simulink model "Per_MKM"  (R2019a)
settings: Solver=FixedStepDiscrete  StartTime=0.0  StopTime=50  FixedStep=1  RelTol=1e-3
undefined symbols (not defined in the file or in its folder): ADAS, ADAS_Setting, KeyPress, Setting
libraries: simulink x102
(part 2 of 2)

== system Per_MKM/Seat_POsitioning_Subsystem/POS_Control5/Subsystem4 ==
  In1 : Inport
  Data Store Read14 : DataStoreRead  DataStoreName=POS_M5
  Data Store Read15 : DataStoreRead  DataStoreName=POS_S15
  Data Store Read16 : DataStoreRead  DataStoreName=POS_S25
  Data Type Conversion : DataTypeConversion
  Multiport Switch3 : MultiPortSwitch  DataPortOrder=Zero-based contiguous  DataPortForDefault=Additional data port  zeroidx=on
  Out1 : Outport
  Out2 : Outport  Port=2
  wires:
  Data Store Read16/1 -> Multiport Switch3/4
  Data Store Read15/1 -> Multiport Switch3/3
  Data Type Conversion/1 -> Multiport Switch3/1
  Multiport Switch3/1 -> Out2/1
  Data Store Read14/1 -> Multiport Switch3/2, Multiport Switch3/5
  In1/1 -> Data Type Conversion/1, Out1/1

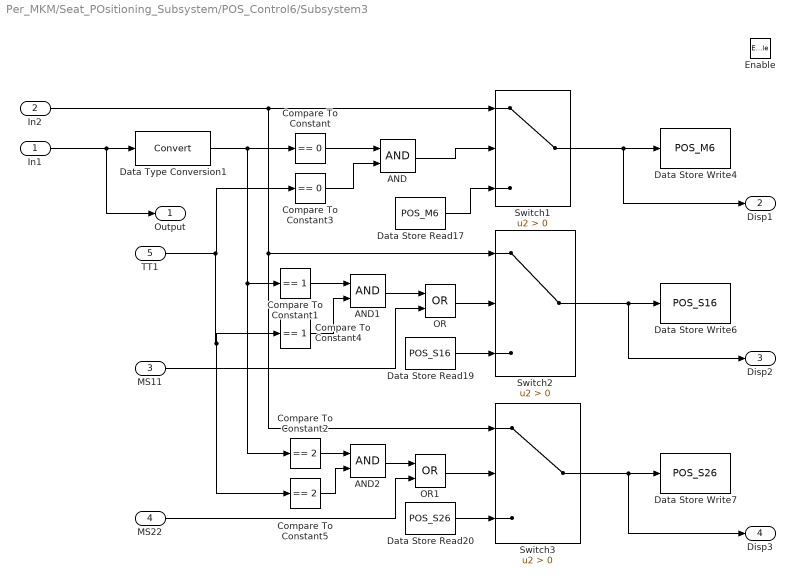
== system Per_MKM/Seat_POsitioning_Subsystem/POS_Control6/Subsystem3 ==
  In1 : Inport
  In2 : Inport  Port=2
  MS11 : Inport  Port=3
  MS22 : Inport  Port=4
  TT1 : Inport  Port=5
  Enable : EnablePort
  AND : Logic  AllPortsSameDT=off  OutDataTypeStr=boolean
  AND1 : Logic  AllPortsSameDT=off  OutDataTypeStr=boolean
  AND2 : Logic  AllPortsSameDT=off  OutDataTypeStr=boolean
  Compare To Constant : simulink/Logic and Bit Operations/Compare To Constant  relop===  const=0  OutDataTypeStr=boolean
  Compare To Constant1 : simulink/Logic and Bit Operations/Compare To Constant  relop===  const=1  OutDataTypeStr=boolean
  Compare To Constant2 : simulink/Logic and Bit Operations/Compare To Constant  relop===  const=2  OutDataTypeStr=boolean
  Compare To Constant3 : simulink/Logic and Bit Operations/Compare To Constant  relop===  const=0  OutDataTypeStr=boolean
  Compare To Constant4 : simulink/Logic and Bit Operations/Compare To Constant  relop===  const=1  OutDataTypeStr=boolean
  Compare To Constant5 : simulink/Logic and Bit Operations/Compare To Constant  relop===  const=2  OutDataTypeStr=boolean
  Data Store Read17 : DataStoreRead  DataStoreName=POS_M6
  Data Store Read19 : DataStoreRead  DataStoreName=POS_S16
  Data Store Read20 : DataStoreRead  DataStoreName=POS_S26
  Data Store Write4 : DataStoreWrite  DataStoreName=POS_M6
  Data Store Write6 : DataStoreWrite  DataStoreName=POS_S16
  Data Store Write7 : DataStoreWrite  DataStoreName=POS_S26
  Data Type Conversion1 : DataTypeConversion
  OR : Logic  Operator=OR  AllPortsSameDT=off  OutDataTypeStr=boolean
  OR1 : Logic  Operator=OR  AllPortsSameDT=off  OutDataTypeStr=boolean
  Switch1 : Switch  Criteria=u2 > Threshold
  Switch2 : Switch  Criteria=u2 > Threshold
  Switch3 : Switch  Criteria=u2 > Threshold
  Output : Outport
  Disp1 : Outport  Port=2
  Disp2 : Outport  Port=3
  Disp3 : Outport  Port=4
  wires:
  Data Type Conversion1/1 -> Compare To Constant/1, Compare To Constant2/1, Compare To Constant1/1
  Switch2/1 -> Disp2/1, Data Store Write6/1
  Data Store Read20/1 -> Switch3/3
  Switch3/1 -> Disp3/1, Data Store Write7/1
  Switch1/1 -> Disp1/1, Data Store Write4/1
  Data Store Read19/1 -> Switch2/3
  Data Store Read17/1 -> Switch1/3
  In1/1 -> Output/1, Data Type Conversion1/1
  In2/1 -> Switch1/1, Switch2/1, Switch3/1
  OR/1 -> Switch2/2
  OR1/1 -> Switch3/2
  MS11/1 -> OR/2
  MS22/1 -> OR1/2
  AND/1 -> Switch1/2
  Compare To Constant/1 -> AND/1
  Compare To Constant3/1 -> AND/2
  TT1/1 -> Compare To Constant5/1, Compare To Constant4/1, Compare To Constant3/1
  Compare To Constant1/1 -> AND1/1
  Compare To Constant4/1 -> AND1/2
  AND1/1 -> OR/1
  AND2/1 -> OR1/1
  Compare To Constant2/1 -> AND2/1
  Compare To Constant5/1 -> AND2/2

== system Per_MKM/Seat_POsitioning_Subsystem/POS_Control6/Subsystem4 ==
  In1 : Inport
  Data Store Read14 : DataStoreRead  DataStoreName=POS_M6
  Data Store Read15 : DataStoreRead  DataStoreName=POS_S16
  Data Store Read16 : DataStoreRead  DataStoreName=POS_S26
  Data Type Conversion : DataTypeConversion
  Multiport Switch3 : MultiPortSwitch  DataPortOrder=Zero-based contiguous  DataPortForDefault=Additional data port  zeroidx=on
  Out1 : Outport
  Out2 : Outport  Port=2
  wires:
  In1/1 -> Out1/1, Data Type Conversion/1
  Data Store Read14/1 -> Multiport Switch3/5, Multiport Switch3/2
  Multiport Switch3/1 -> Out2/1
  Data Type Conversion/1 -> Multiport Switch3/1
  Data Store Read15/1 -> Multiport Switch3/3
  Data Store Read16/1 -> Multiport Switch3/4

== system Per_MKM/Subsystem2/Subsystem/Subsystem_ACC ==
  In1 : Inport
  ACC2 : simulink/Sources/Enumerated Constant  OutDataTypeStr=Enum: ADAS  Value=ADAS.Adaptive_Cruse_Control_Enable  SampleTime=inf
      settings: SourceProductName=Simulink
  ACC3 : simulink/Sources/Enumerated Constant  OutDataTypeStr=Enum: ADAS  Value=ADAS.Adaptive_Cruse_Control_Disable  SampleTime=inf
      settings: SourceProductName=Simulink
  ACC4 : simulink/Sources/Enumerated Constant  OutDataTypeStr=Enum: ADAS  Value=ADAS.Disable  SampleTime=inf
      settings: SourceProductName=Simulink
  Data Store Read1 : DataStoreRead  DataStoreName=ADAS_M
  Data Store Read2 : DataStoreRead  DataStoreName=ADAS_S1
  Data Store Read3 : DataStoreRead  DataStoreName=ADAS_S2
  Data Type Conversion{2..6} (5 alike) : DataTypeConversion
  Enumerated Constant : simulink/Sources/Enumerated Constant  OutDataTypeStr=Enum: KeyPress  Value=KeyPress.No_User  SampleTime=inf
      settings: SourceProductName=Simulink
  Multiport Switch : MultiPortSwitch
  Multiport Switch1 : MultiPortSwitch  DataPortOrder=Zero-based contiguous  Inputs=4  zeroidx=on
  Out1 : Outport
  wires:
  ACC4/1 -> Multiport Switch/4
  Data Store Read3/1 -> Data Type Conversion5/1
  Data Type Conversion4/1 -> Multiport Switch1/3
  ACC3/1 -> Multiport Switch/3
  Data Store Read1/1 -> Data Type Conversion3/1
  Multiport Switch1/1 -> Multiport Switch/1
  ACC2/1 -> Multiport Switch/2
  In1/1 -> Data Type Conversion2/1
  Data Store Read2/1 -> Data Type Conversion4/1
  Enumerated Constant/1 -> Data Type Conversion6/1
  Data Type Conversion2/1 -> Multiport Switch1/1
  Data Type Conversion5/1 -> Multiport Switch1/4
  Data Type Conversion3/1 -> Multiport Switch1/2
  Data Type Conversion6/1 -> Multiport Switch1/5
  Multiport Switch/1 -> Out1/1

== system Per_MKM/Subsystem2/Subsystem/Subsystem_APSD ==
  In1 : Inport
  ACC2 : simulink/Sources/Enumerated Constant  OutDataTypeStr=Enum: ADAS  Value=ADAS.Automatic_Parking_System_Enable  SampleTime=inf
      settings: SourceProductName=Simulink
  ACC3 : simulink/Sources/Enumerated Constant  OutDataTypeStr=Enum: ADAS  Value=ADAS.Automatic_Parking_System_Disable  SampleTime=inf
      settings: SourceProductName=Simulink
  ACC4 : simulink/Sources/Enumerated Constant  OutDataTypeStr=Enum: ADAS  Value=ADAS.Disable  SampleTime=inf
      settings: SourceProductName=Simulink
  Data Store Read1 : DataStoreRead  DataStoreName=ADAS_M2
  Data Store Read2 : DataStoreRead  DataStoreName=ADAS_S12
  Data Store Read3 : DataStoreRead  DataStoreName=ADAS_S22
  Data Type Conversion{2..6} (5 alike) : DataTypeConversion
  Enumerated Constant : simulink/Sources/Enumerated Constant  OutDataTypeStr=Enum: KeyPress  Value=KeyPress.No_User  SampleTime=inf
      settings: SourceProductName=Simulink
  Multiport Switch : MultiPortSwitch
  Multiport Switch1 : MultiPortSwitch  DataPortOrder=Zero-based contiguous  Inputs=4  zeroidx=on
  Out1 : Outport
  wires:
  Data Store Read2/1 -> Data Type Conversion4/1
  ACC2/1 -> Multiport Switch/2
  Enumerated Constant/1 -> Data Type Conversion6/1
  ACC3/1 -> Multiport Switch/3
  Data Type Conversion2/1 -> Multiport Switch1/1
  Data Type Conversion4/1 -> Multiport Switch1/3
  Data Type Conversion6/1 -> Multiport Switch1/5
  Data Store Read3/1 -> Data Type Conversion5/1
  ACC4/1 -> Multiport Switch/4
  Data Type Conversion3/1 -> Multiport Switch1/2
  Data Type Conversion5/1 -> Multiport Switch1/4
  Data Store Read1/1 -> Data Type Conversion3/1
  Multiport Switch1/1 -> Multiport Switch/1
  In1/1 -> Data Type Conversion2/1
  Multiport Switch/1 -> Out1/1

== system Per_MKM/Subsystem2/Subsystem/Subsystem_DDDE ==
  In1 : Inport
  ACC2 : simulink/Sources/Enumerated Constant  OutDataTypeStr=Enum: ADAS  Value=ADAS.Driver_Drowsiness_detection_Enable  SampleTime=inf
      settings: SourceProductName=Simulink
  ACC3 : simulink/Sources/Enumerated Constant  OutDataTypeStr=Enum: ADAS  Value=ADAS.Driver_Drowsiness_detection_Disable  SampleTime=inf
      settings: SourceProductName=Simulink
  ACC4 : simulink/Sources/Enumerated Constant  OutDataTypeStr=Enum: ADAS  Value=ADAS.Disable  SampleTime=inf
      settings: SourceProductName=Simulink
  Data Store Read1 : DataStoreRead  DataStoreName=ADAS_M1
  Data Store Read2 : DataStoreRead  DataStoreName=ADAS_S11
  Data Store Read3 : DataStoreRead  DataStoreName=ADAS_S21
  Data Type Conversion{2..6} (5 alike) : DataTypeConversion
  Enumerated Constant : simulink/Sources/Enumerated Constant  OutDataTypeStr=Enum: KeyPress  Value=KeyPress.No_User  SampleTime=inf
      settings: SourceProductName=Simulink
  Multiport Switch : MultiPortSwitch
  Multiport Switch1 : MultiPortSwitch  DataPortOrder=Zero-based contiguous  Inputs=4  zeroidx=on
  Out1 : Outport
  wires:
  Enumerated Constant/1 -> Data Type Conversion6/1
  Data Store Read3/1 -> Data Type Conversion5/1
  Data Store Read1/1 -> Data Type Conversion3/1
  ACC4/1 -> Multiport Switch/4
  Multiport Switch1/1 -> Multiport Switch/1
  ACC3/1 -> Multiport Switch/3
  Data Type Conversion6/1 -> Multiport Switch1/5
  Data Type Conversion5/1 -> Multiport Switch1/4
  Data Type Conversion3/1 -> Multiport Switch1/2
  Data Type Conversion2/1 -> Multiport Switch1/1
  Data Store Read2/1 -> Data Type Conversion4/1
  Data Type Conversion4/1 -> Multiport Switch1/3
  ACC2/1 -> Multiport Switch/2
  In1/1 -> Data Type Conversion2/1
  Multiport Switch/1 -> Out1/1

== system Per_MKM/Subsystem2/Subsystem/Subsystem_TSRC ==
  In1 : Inport
  ACC2 : simulink/Sources/Enumerated Constant  OutDataTypeStr=Enum: ADAS  Value=ADAS.Trafic_Signal_Recognization_Enable  SampleTime=inf
      settings: SourceProductName=Simulink
  ACC3 : simulink/Sources/Enumerated Constant  OutDataTypeStr=Enum: ADAS  Value=ADAS.Trafic_Signal_Recognization_Disable  SampleTime=inf
      settings: SourceProductName=Simulink
  ACC4 : simulink/Sources/Enumerated Constant  OutDataTypeStr=Enum: ADAS  Value=ADAS.Disable  SampleTime=inf
      settings: SourceProductName=Simulink
  Data Store Read1 : DataStoreRead  DataStoreName=ADAS_M3
  Data Store Read2 : DataStoreRead  DataStoreName=ADAS_S13
  Data Store Read3 : DataStoreRead  DataStoreName=ADAS_S23
  Data Type Conversion{2..6} (5 alike) : DataTypeConversion
  Enumerated Constant : simulink/Sources/Enumerated Constant  OutDataTypeStr=Enum: KeyPress  Value=KeyPress.No_User  SampleTime=inf
      settings: SourceProductName=Simulink
  Multiport Switch : MultiPortSwitch
  Multiport Switch1 : MultiPortSwitch  DataPortOrder=Zero-based contiguous  Inputs=4  zeroidx=on
  Out1 : Outport
  wires:
  ACC4/1 -> Multiport Switch/4
  Data Type Conversion2/1 -> Multiport Switch1/1
  Data Type Conversion5/1 -> Multiport Switch1/4
  Data Store Read2/1 -> Data Type Conversion4/1
  Data Store Read3/1 -> Data Type Conversion5/1
  Data Type Conversion4/1 -> Multiport Switch1/3
  Enumerated Constant/1 -> Data Type Conversion6/1
  Data Type Conversion6/1 -> Multiport Switch1/5
  ACC2/1 -> Multiport Switch/2
  ACC3/1 -> Multiport Switch/3
  Data Store Read1/1 -> Data Type Conversion3/1
  Data Type Conversion3/1 -> Multiport Switch1/2
  Multiport Switch1/1 -> Multiport Switch/1
  In1/1 -> Data Type Conversion2/1
  Multiport Switch/1 -> Out1/1

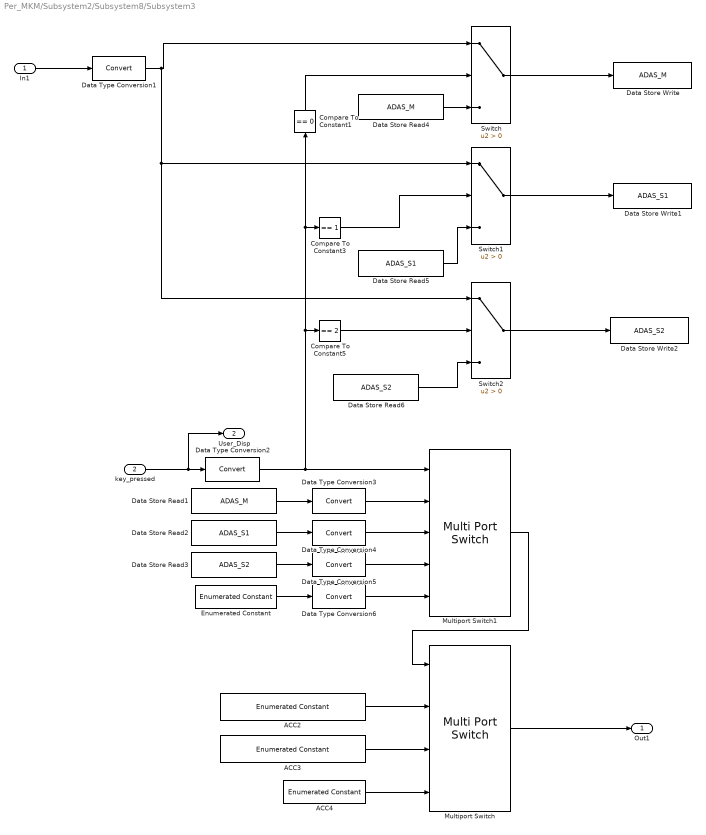
== system Per_MKM/Subsystem2/Subsystem8/Subsystem3 ==
  In1 : Inport
  key_pressed : Inport  Port=2
  ACC2 : simulink/Sources/Enumerated Constant  OutDataTypeStr=Enum: ADAS  Value=ADAS.Adaptive_Cruse_Control_Enable  SampleTime=inf
      settings: SourceProductName=Simulink
  ACC3 : simulink/Sources/Enumerated Constant  OutDataTypeStr=Enum: ADAS  Value=ADAS.Adaptive_Cruse_Control_Disable  SampleTime=inf
      settings: SourceProductName=Simulink
  ACC4 : simulink/Sources/Enumerated Constant  OutDataTypeStr=Enum: ADAS  Value=ADAS.Disable  SampleTime=inf
      settings: SourceProductName=Simulink
  Compare To Constant1 : simulink/Logic and Bit Operations/Compare To Constant  relop===  const=0  OutDataTypeStr=boolean
  Compare To Constant3 : simulink/Logic and Bit Operations/Compare To Constant  relop===  const=1  OutDataTypeStr=boolean
  Compare To Constant5 : simulink/Logic and Bit Operations/Compare To Constant  relop===  const=2  OutDataTypeStr=boolean
  Data Store Read1 : DataStoreRead  DataStoreName=ADAS_M
  Data Store Read2 : DataStoreRead  DataStoreName=ADAS_S1
  Data Store Read3 : DataStoreRead  DataStoreName=ADAS_S2
  Data Store Read4 : DataStoreRead  DataStoreName=ADAS_M
  Data Store Read5 : DataStoreRead  DataStoreName=ADAS_S1
  Data Store Read6 : DataStoreRead  DataStoreName=ADAS_S2
  Data Store Write : DataStoreWrite  DataStoreName=ADAS_M
  Data Store Write1 : DataStoreWrite  DataStoreName=ADAS_S1
  Data Store Write2 : DataStoreWrite  DataStoreName=ADAS_S2
  Data Type Conversion{1..6} (6 alike) : DataTypeConversion
  Enumerated Constant : simulink/Sources/Enumerated Constant  OutDataTypeStr=Enum: KeyPress  Value=KeyPress.No_User  SampleTime=inf
      settings: SourceProductName=Simulink
  Multiport Switch : MultiPortSwitch
  Multiport Switch1 : MultiPortSwitch  DataPortOrder=Zero-based contiguous  Inputs=4  zeroidx=on
  Switch : Switch  Criteria=u2 > Threshold
  Switch1 : Switch  Criteria=u2 > Threshold
  Switch2 : Switch  Criteria=u2 > Threshold
  Out1 : Outport
  User_Disp : Outport  Port=2
  wires:
  Data Store Read6/1 -> Switch2/3
  Switch2/1 -> Data Store Write2/1
  Compare To Constant5/1 -> Switch2/2
  Data Store Read5/1 -> Switch1/3
  Switch1/1 -> Data Store Write1/1
  Data Type Conversion1/1 -> Switch/1, Switch1/1, Switch2/1
  Compare To Constant3/1 -> Switch1/2
  Compare To Constant1/1 -> Switch/2
  Data Type Conversion6/1 -> Multiport Switch1/5
  Data Type Conversion5/1 -> Multiport Switch1/4
  Data Type Conversion4/1 -> Multiport Switch1/3
  Data Type Conversion3/1 -> Multiport Switch1/2
  Multiport Switch1/1 -> Multiport Switch/1
  Enumerated Constant/1 -> Data Type Conversion6/1
  Data Store Read3/1 -> Data Type Conversion5/1
  Data Store Read2/1 -> Data Type Conversion4/1
  Data Store Read1/1 -> Data Type Conversion3/1
  Data Type Conversion2/1 -> Multiport Switch1/1, Compare To Constant5/1, Compare To Constant3/1, Compare To Constant1/1
  key_pressed/1 -> Data Type Conversion2/1, User_Disp/1
  Multiport Switch/1 -> Out1/1
  In1/1 -> Data Type Conversion1/1
  Switch/1 -> Data Store Write/1
  ACC4/1 -> Multiport Switch/4
  ACC2/1 -> Multiport Switch/2
  Data Store Read4/1 -> Switch/3
  ACC3/1 -> Multiport Switch/3

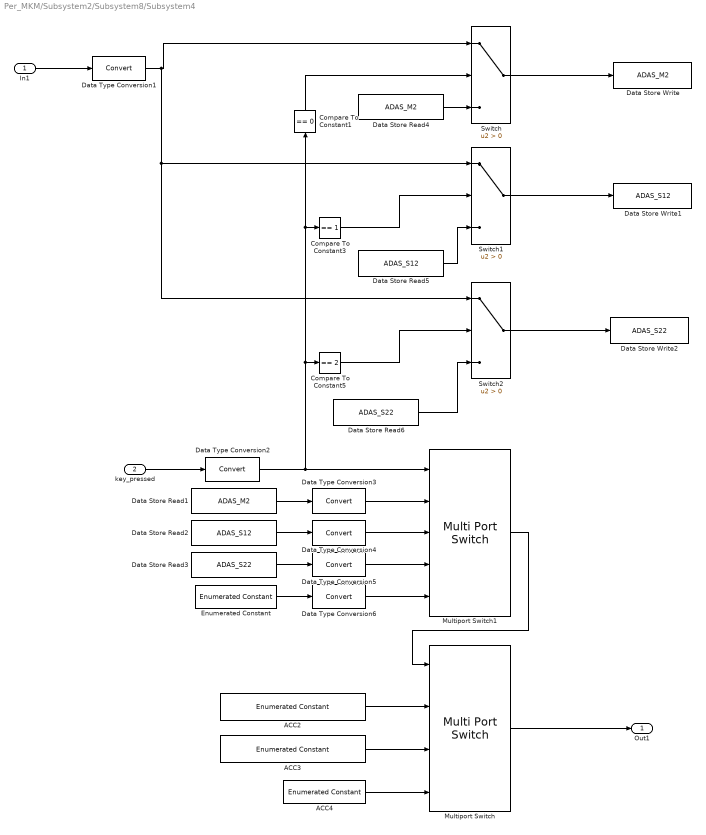
== system Per_MKM/Subsystem2/Subsystem8/Subsystem4 ==
  In1 : Inport
  key_pressed : Inport  Port=2
  ACC2 : simulink/Sources/Enumerated Constant  OutDataTypeStr=Enum: ADAS  Value=ADAS.Automatic_Parking_System_Enable  SampleTime=inf
      settings: SourceProductName=Simulink
  ACC3 : simulink/Sources/Enumerated Constant  OutDataTypeStr=Enum: ADAS  Value=ADAS.Automatic_Parking_System_Disable  SampleTime=inf
      settings: SourceProductName=Simulink
  ACC4 : simulink/Sources/Enumerated Constant  OutDataTypeStr=Enum: ADAS  Value=ADAS.Disable  SampleTime=inf
      settings: SourceProductName=Simulink
  Compare To Constant1 : simulink/Logic and Bit Operations/Compare To Constant  relop===  const=0  OutDataTypeStr=boolean
  Compare To Constant3 : simulink/Logic and Bit Operations/Compare To Constant  relop===  const=1  OutDataTypeStr=boolean
  Compare To Constant5 : simulink/Logic and Bit Operations/Compare To Constant  relop===  const=2  OutDataTypeStr=boolean
  Data Store Read1 : DataStoreRead  DataStoreName=ADAS_M2
  Data Store Read2 : DataStoreRead  DataStoreName=ADAS_S12
  Data Store Read3 : DataStoreRead  DataStoreName=ADAS_S22
  Data Store Read4 : DataStoreRead  DataStoreName=ADAS_M2
  Data Store Read5 : DataStoreRead  DataStoreName=ADAS_S12
  Data Store Read6 : DataStoreRead  DataStoreName=ADAS_S22
  Data Store Write : DataStoreWrite  DataStoreName=ADAS_M2
  Data Store Write1 : DataStoreWrite  DataStoreName=ADAS_S12
  Data Store Write2 : DataStoreWrite  DataStoreName=ADAS_S22
  Data Type Conversion{1..6} (6 alike) : DataTypeConversion
  Enumerated Constant : simulink/Sources/Enumerated Constant  OutDataTypeStr=Enum: KeyPress  Value=KeyPress.No_User  SampleTime=inf
      settings: SourceProductName=Simulink
  Multiport Switch : MultiPortSwitch
  Multiport Switch1 : MultiPortSwitch  DataPortOrder=Zero-based contiguous  Inputs=4  zeroidx=on
  Switch : Switch  Criteria=u2 > Threshold
  Switch1 : Switch  Criteria=u2 > Threshold
  Switch2 : Switch  Criteria=u2 > Threshold
  Out1 : Outport
  wires:
  Data Store Read6/1 -> Switch2/3
  Switch2/1 -> Data Store Write2/1
  Compare To Constant5/1 -> Switch2/2
  Data Store Read5/1 -> Switch1/3
  Switch1/1 -> Data Store Write1/1
  Data Type Conversion1/1 -> Switch/1, Switch1/1, Switch2/1
  Compare To Constant3/1 -> Switch1/2
  Compare To Constant1/1 -> Switch/2
  Data Type Conversion6/1 -> Multiport Switch1/5
  Data Type Conversion5/1 -> Multiport Switch1/4
  Data Type Conversion4/1 -> Multiport Switch1/3
  Data Type Conversion3/1 -> Multiport Switch1/2
  Multiport Switch1/1 -> Multiport Switch/1
  Enumerated Constant/1 -> Data Type Conversion6/1
  Data Store Read3/1 -> Data Type Conversion5/1
  Data Store Read2/1 -> Data Type Conversion4/1
  Data Store Read1/1 -> Data Type Conversion3/1
  Data Type Conversion2/1 -> Multiport Switch1/1, Compare To Constant5/1, Compare To Constant3/1, Compare To Constant1/1
  key_pressed/1 -> Data Type Conversion2/1
  Multiport Switch/1 -> Out1/1
  In1/1 -> Data Type Conversion1/1
  Switch/1 -> Data Store Write/1
  ACC4/1 -> Multiport Switch/4
  ACC2/1 -> Multiport Switch/2
  Data Store Read4/1 -> Switch/3
  ACC3/1 -> Multiport Switch/3

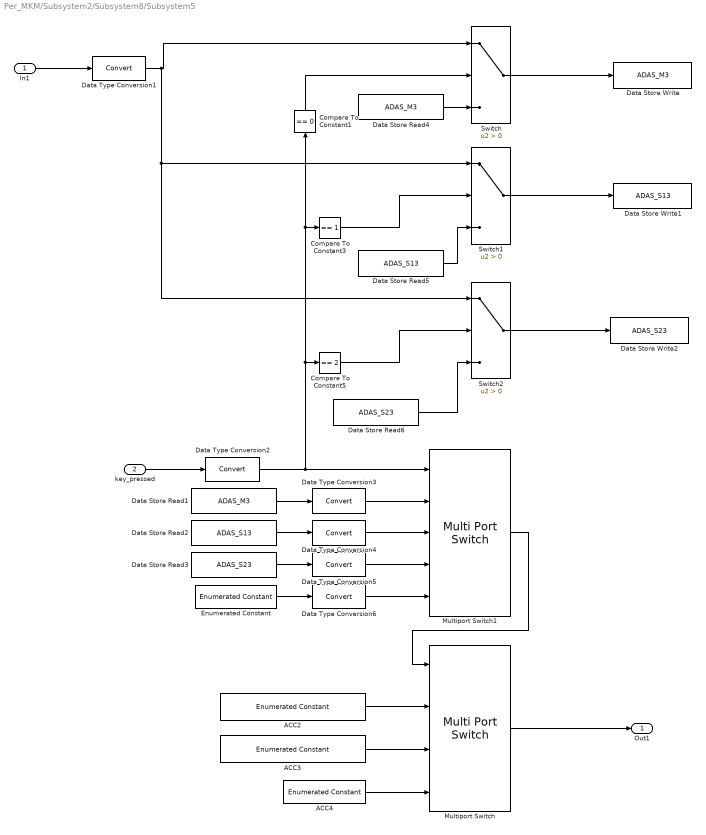
== system Per_MKM/Subsystem2/Subsystem8/Subsystem5 ==
  In1 : Inport
  key_pressed : Inport  Port=2
  ACC2 : simulink/Sources/Enumerated Constant  OutDataTypeStr=Enum: ADAS  Value=ADAS.Trafic_Signal_Recognization_Enable  SampleTime=inf
      settings: SourceProductName=Simulink
  ACC3 : simulink/Sources/Enumerated Constant  OutDataTypeStr=Enum: ADAS  Value=ADAS.Trafic_Signal_Recognization_Disable  SampleTime=inf
      settings: SourceProductName=Simulink
  ACC4 : simulink/Sources/Enumerated Constant  OutDataTypeStr=Enum: ADAS  Value=ADAS.Disable  SampleTime=inf
      settings: SourceProductName=Simulink
  Compare To Constant1 : simulink/Logic and Bit Operations/Compare To Constant  relop===  const=0  OutDataTypeStr=boolean
  Compare To Constant3 : simulink/Logic and Bit Operations/Compare To Constant  relop===  const=1  OutDataTypeStr=boolean
  Compare To Constant5 : simulink/Logic and Bit Operations/Compare To Constant  relop===  const=2  OutDataTypeStr=boolean
  Data Store Read1 : DataStoreRead  DataStoreName=ADAS_M3
  Data Store Read2 : DataStoreRead  DataStoreName=ADAS_S13
  Data Store Read3 : DataStoreRead  DataStoreName=ADAS_S23
  Data Store Read4 : DataStoreRead  DataStoreName=ADAS_M3
  Data Store Read5 : DataStoreRead  DataStoreName=ADAS_S13
  Data Store Read6 : DataStoreRead  DataStoreName=ADAS_S23
  Data Store Write : DataStoreWrite  DataStoreName=ADAS_M3
  Data Store Write1 : DataStoreWrite  DataStoreName=ADAS_S13
  Data Store Write2 : DataStoreWrite  DataStoreName=ADAS_S23
  Data Type Conversion{1..6} (6 alike) : DataTypeConversion
  Enumerated Constant : simulink/Sources/Enumerated Constant  OutDataTypeStr=Enum: KeyPress  Value=KeyPress.No_User  SampleTime=inf
      settings: SourceProductName=Simulink
  Multiport Switch : MultiPortSwitch
  Multiport Switch1 : MultiPortSwitch  DataPortOrder=Zero-based contiguous  Inputs=4  zeroidx=on
  Switch : Switch  Criteria=u2 > Threshold
  Switch1 : Switch  Criteria=u2 > Threshold
  Switch2 : Switch  Criteria=u2 > Threshold
  Out1 : Outport
  wires:
  ACC3/1 -> Multiport Switch/3
  Data Store Read4/1 -> Switch/3
  ACC2/1 -> Multiport Switch/2
  ACC4/1 -> Multiport Switch/4
  Switch/1 -> Data Store Write/1
  In1/1 -> Data Type Conversion1/1
  Multiport Switch/1 -> Out1/1
  key_pressed/1 -> Data Type Conversion2/1
  Data Type Conversion2/1 -> Compare To Constant1/1, Compare To Constant3/1, Compare To Constant5/1, Multiport Switch1/1
  Data Store Read1/1 -> Data Type Conversion3/1
  Data Store Read2/1 -> Data Type Conversion4/1
  Data Store Read3/1 -> Data Type Conversion5/1
  Enumerated Constant/1 -> Data Type Conversion6/1
  Multiport Switch1/1 -> Multiport Switch/1
  Data Type Conversion3/1 -> Multiport Switch1/2
  Data Type Conversion4/1 -> Multiport Switch1/3
  Data Type Conversion5/1 -> Multiport Switch1/4
  Data Type Conversion6/1 -> Multiport Switch1/5
  Compare To Constant1/1 -> Switch/2
  Compare To Constant3/1 -> Switch1/2
  Data Type Conversion1/1 -> Switch2/1, Switch1/1, Switch/1
  Switch1/1 -> Data Store Write1/1
  Data Store Read5/1 -> Switch1/3
  Compare To Constant5/1 -> Switch2/2
  Switch2/1 -> Data Store Write2/1
  Data Store Read6/1 -> Switch2/3

== system Per_MKM/Subsystem2/Subsystem8/Subsystem7 ==
  In1 : Inport
  key_pressed : Inport  Port=2
  ACC2 : simulink/Sources/Enumerated Constant  OutDataTypeStr=Enum: ADAS  Value=ADAS.Driver_Drowsiness_detection_Enable  SampleTime=inf
      settings: SourceProductName=Simulink
  ACC3 : simulink/Sources/Enumerated Constant  OutDataTypeStr=Enum: ADAS  Value=ADAS.Driver_Drowsiness_detection_Disable  SampleTime=inf
      settings: SourceProductName=Simulink
  ACC4 : simulink/Sources/Enumerated Constant  OutDataTypeStr=Enum: ADAS  Value=ADAS.Disable  SampleTime=inf
      settings: SourceProductName=Simulink
  Compare To Constant1 : simulink/Logic and Bit Operations/Compare To Constant  relop===  const=0  OutDataTypeStr=boolean
  Compare To Constant3 : simulink/Logic and Bit Operations/Compare To Constant  relop===  const=1  OutDataTypeStr=boolean
  Compare To Constant5 : simulink/Logic and Bit Operations/Compare To Constant  relop===  const=2  OutDataTypeStr=boolean
  Data Store Read1 : DataStoreRead  DataStoreName=ADAS_M1
  Data Store Read2 : DataStoreRead  DataStoreName=ADAS_S11
  Data Store Read3 : DataStoreRead  DataStoreName=ADAS_S21
  Data Store Read4 : DataStoreRead  DataStoreName=ADAS_M1
  Data Store Read5 : DataStoreRead  DataStoreName=ADAS_S11
  Data Store Read6 : DataStoreRead  DataStoreName=ADAS_S21
  Data Store Write : DataStoreWrite  DataStoreName=ADAS_M1
  Data Store Write1 : DataStoreWrite  DataStoreName=ADAS_S11
  Data Store Write2 : DataStoreWrite  DataStoreName=ADAS_S21
  Data Type Conversion{1..6} (6 alike) : DataTypeConversion
  Enumerated Constant : simulink/Sources/Enumerated Constant  OutDataTypeStr=Enum: KeyPress  Value=KeyPress.No_User  SampleTime=inf
      settings: SourceProductName=Simulink
  Multiport Switch : MultiPortSwitch
  Multiport Switch1 : MultiPortSwitch  DataPortOrder=Zero-based contiguous  Inputs=4  zeroidx=on
  Switch : Switch  Criteria=u2 > Threshold
  Switch1 : Switch  Criteria=u2 > Threshold
  Switch2 : Switch  Criteria=u2 > Threshold
  Out1 : Outport
  wires:
  ACC3/1 -> Multiport Switch/3
  Data Store Read4/1 -> Switch/3
  ACC2/1 -> Multiport Switch/2
  ACC4/1 -> Multiport Switch/4
  Switch/1 -> Data Store Write/1
  In1/1 -> Data Type Conversion1/1
  Multiport Switch/1 -> Out1/1
  key_pressed/1 -> Data Type Conversion2/1
  Data Type Conversion2/1 -> Compare To Constant1/1, Compare To Constant3/1, Compare To Constant5/1, Multiport Switch1/1
  Data Store Read1/1 -> Data Type Conversion3/1
  Data Store Read2/1 -> Data Type Conversion4/1
  Data Store Read3/1 -> Data Type Conversion5/1
  Enumerated Constant/1 -> Data Type Conversion6/1
  Multiport Switch1/1 -> Multiport Switch/1
  Data Type Conversion3/1 -> Multiport Switch1/2
  Data Type Conversion4/1 -> Multiport Switch1/3
  Data Type Conversion5/1 -> Multiport Switch1/4
  Data Type Conversion6/1 -> Multiport Switch1/5
  Compare To Constant1/1 -> Switch/2
  Compare To Constant3/1 -> Switch1/2
  Data Type Conversion1/1 -> Switch2/1, Switch1/1, Switch/1
  Switch1/1 -> Data Store Write1/1
  Data Store Read5/1 -> Switch1/3
  Compare To Constant5/1 -> Switch2/2
  Switch2/1 -> Data Store Write2/1
  Data Store Read6/1 -> Switch2/3
